simulink model "model2v1"  (R2020b)
settings: Solver=VariableStepAuto  StartTime=0.0  StopTime=10.0  RelTol=1e-3
settings Model: Creator=dkravchenko  LastModifiedBy=dkravchenko

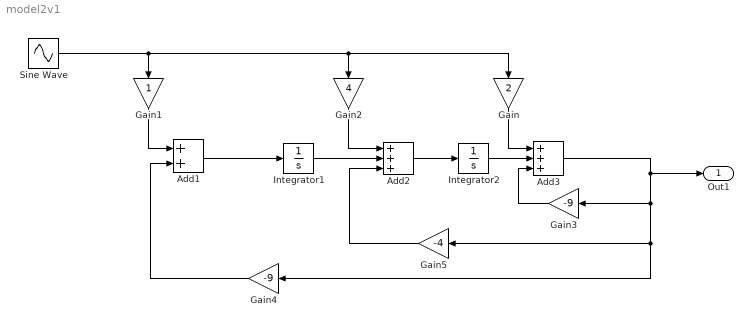
== system model2v1 ==
  Add1 : Sum
  Add2 : Sum  Inputs=+++
  Add3 : Sum  Inputs=+++
  Gain : Gain  Gain=2
  Gain1 : Gain
  Gain2 : Gain  Gain=4
  Gain3 : Gain  Gain=-9
  Gain4 : Gain  Gain=-9
  Gain5 : Gain  Gain=-4
  Integrator1 : Integrator  InitialCondition=18.5
  Integrator2 : Integrator  InitialCondition=5
  Sine Wave : Sin  Amplitude=0  SampleTime=0
  Out1 : Outport
  wires:
  Gain4/1 -> Add1/2
  Sine Wave/1 -> Gain/1, Gain2/1, Gain1/1
  Gain2/1 -> Add2/1
  Integrator1/1 -> Add2/2
  Gain1/1 -> Add1/1
  Gain/1 -> Add3/1
  Gain5/1 -> Add2/3
  Add3/1 -> Out1/1, Gain3/1, Gain4/1, Gain5/1
  Add2/1 -> Integrator2/1
  Integrator2/1 -> Add3/2
  Add1/1 -> Integrator1/1
  Gain3/1 -> Add3/3
